simulink model "nmm2DFullBody"  (R2018a)
settings: Solver=ode23s  StartTime=0.0  StopTime=13  FixedStep=1e-3  MaxStep=ts_max  RelTol=1e-3  AbsTol=1e-4  EnableMultiTasking=on
InitFcn:
  | addpath('../lib');
  | addpath('./init_script');
  | nms_model_MechInit
  | nms_model_ControlInit
StopFcn:
  | mRFX = struct;
  | 
  | mRFX.RStance = DataFromModel.Data(:,2)
  | mRFX.RGRF_AP = DataFromModel.Data(:,24)
  | mRFX.RGRF_VT = DataFromModel.Data(:,22)
  | mRFX.RAnkleAngle = DataFromModel.Data(:,8)
  | mRFX.RKneeAngle = DataFromModel.Data(:,7)
  | mRFX.RHipAngle = DataFromModel.Data(:,6)
  | mRFX.RAnkleTorque = DataFromModel.Data(:,20)
  | mRFX.RKneeTorque = DataFromModel.Data(:,19)
  | mRFX.RHipTorque = DataFromModel.Data(:,18)
  | 
  | mRFX.RMuscleGLU = DataFromModel.Data(:,32)
  | mRFX.RMuscleHF = DataFromModel.Data(:,33)
  | mRFX.RMuscleHAM = DataFromModel.Data(:,34)
  | mRFX.RMuscleVAS = DataFromModel.Data(:,35)
  | mRFX.RMuscleGAS = DataFromModel.Data(:,36)
  | mRFX.RMuscleSOL = DataFromModel.Data(:,37)
  | mRFX.RMuscleTA = DataFromModel.Data(:,38)
  | 
  | mRFX.LStance = DataFromModel.Data(:,1)
  | mRFX.LGRF_AP = DataFromModel.Data(:,23)
  | mRFX.LGRF_VT = DataFromModel.Data(:,21)
  | mRFX.LAnkleAngle = DataFromModel.Data(:,5)
  | mRFX.LKneeAngle = DataFromModel.Data(:,4)
  | mRFX.LHipAngle = DataFromModel.Data(:,3)
  | mRFX.LAnkleTorque = DataFromModel.Data(:,17)
  | mRFX.LKneeTorque = DataFromModel.Data(:,16)
  | mRFX.LHipTorque = DataFromModel.Data(:,15)
  | 
  | mRFX.LMuscleGLU = DataFromModel.Data(:,25)
  | mRFX.LMuscleHF = DataFromModel.Data(:,26)
  | mRFX.LMuscleHAM = DataFromModel.Data(:,27)
  | mRFX.LMuscleVAS = DataFromModel.Data(:,28)
  | mRFX.LMuscleGAS = DataFromModel.Data(:,29)
  | mRFX.LMuscleSOL = DataFromModel.Data(:,30)
  | mRFX.LMuscleTA = DataFromModel.Data(:,31)
undefined symbols (not defined in the file or in its folder): alphaFmGas, alphaFmGlu, alphaFmHam, alphaFmSol, alphaFmVas, alphaLceHam, alphaLceHfl, alphaLceTa, alphaLceTa1, Amp, amp_var, c, c_jointstop, D12_F, D12_S, D12_T, D13_F, D1G_F, D1G_HAT, D1G_S, D1G_T, DeltaThRef, eref, FmaxGAS, FmaxGLU, FmaxHAM, FmaxHFL, FmaxSOL, FmaxTA, FmaxVAS, freq, freq_var, GainDeltaTheta, GainGAS, GainGLU, GainHAM, GainHAMHFL, GainHFL, GainKneOverExt, GainSOL, GainSOLTA, GainTA, GainVAS, In_F, In_HAT, In_S, In_T, K, k_gx, k_gy, k_pressure, K_swing, LceOffsetHAM, LceOffsetHFL, LceOffsetTA, LongDelay, loptGAS, loptGLU, loptHAM, loptHFL ... (+83)
libraries: nmc x77, mblibv1 x60, simulink x33, simulink_extras x18
(part 6 of 8)

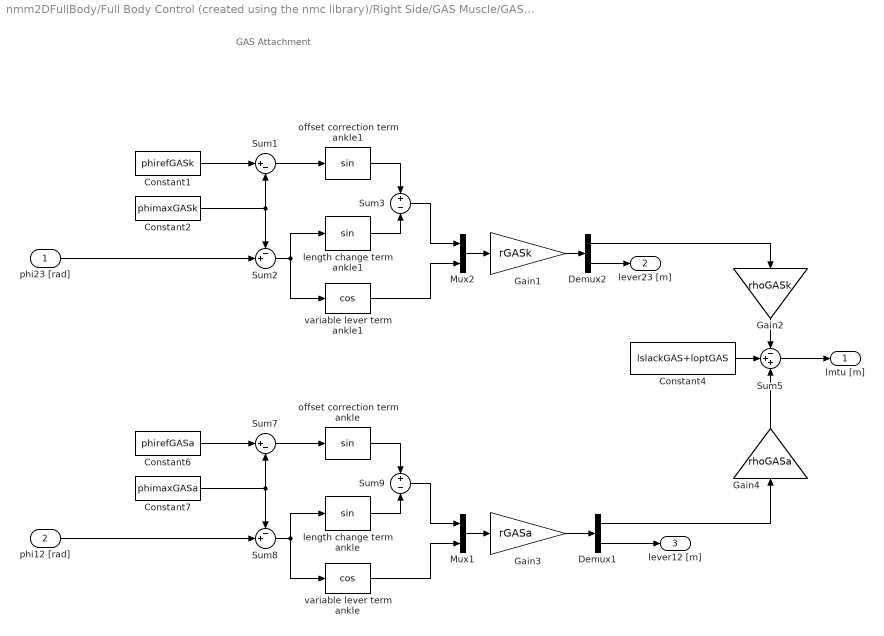
== system nmm2DFullBody/Full Body Control (created using the nmc library)/Right Side/GAS Muscle/GAS Actuation /GAS Link ==
  note: GAS Attachment
  phi23 [rad] : Inport
  phi12 [rad] : Inport  Port=2
  Constant1 : Constant  Value=phirefGASk
  Constant2 : Constant  Value=phimaxGASk
  Constant4 : Constant  Value=lslackGAS+loptGAS
  Constant6 : Constant  Value=phirefGASa
  Constant7 : Constant  Value=phimaxGASa
  Demux1 : Demux  Outputs=2
  Demux2 : Demux  Outputs=2
  Gain1 : Gain  Gain=rGASk
  Gain2 : Gain  Gain=rhoGASk
  Gain3 : Gain  Gain=rGASa
  Gain4 : Gain  Gain=rhoGASa
  Mux1 : Mux  Inputs=2
  Mux2 : Mux  Inputs=2
  Sum1 : Sum  Inputs=|+-
  Sum2 : Sum  Inputs=-+|
  Sum3 : Sum  Inputs=+-
  Sum5 : Sum  Inputs=-++
  Sum7 : Sum  Inputs=|+-
  Sum8 : Sum  Inputs=-+|
  Sum9 : Sum  Inputs=+-
  length change term ankle : Trigonometry
  length change term ankle1 : Trigonometry
  offset correction term ankle : Trigonometry
  offset correction term ankle1 : Trigonometry
  variable lever term ankle : Trigonometry  Operator=cos
  variable lever term ankle1 : Trigonometry  Operator=cos
  lmtu [m] : Outport
  lever23 [m] : Outport  Port=2
  lever12 [m] : Outport  Port=3
  wires:
  phi12 [rad]/1 -> Sum8/2
  Sum5/1 -> lmtu [m]/1
  variable lever term ankle/1 -> Mux1/2
  Demux1/2 -> lever12 [m]/1
  Sum8/1 -> variable lever term ankle/1, length change term ankle/1
  Constant7/1 -> Sum8/1, Sum7/2
  Sum7/1 -> offset correction term ankle/1
  Constant6/1 -> Sum7/1
  length change term ankle/1 -> Sum9/2
  offset correction term ankle/1 -> Sum9/1
  Sum9/1 -> Mux1/1
  Constant4/1 -> Sum5/2
  Mux1/1 -> Gain3/1
  Gain3/1 -> Demux1/1
  Demux1/1 -> Gain4/1
  Gain4/1 -> Sum5/3
  phi23 [rad]/1 -> Sum2/2
  variable lever term ankle1/1 -> Mux2/2
  Sum2/1 -> variable lever term ankle1/1, length change term ankle1/1
  Constant2/1 -> Sum2/1, Sum1/2
  Sum1/1 -> offset correction term ankle1/1
  Constant1/1 -> Sum1/1
  length change term ankle1/1 -> Sum3/2
  offset correction term ankle1/1 -> Sum3/1
  Sum3/1 -> Mux2/1
  Mux2/1 -> Gain1/1
  Gain1/1 -> Demux2/1
  Demux2/2 -> lever23 [m]/1
  Demux2/1 -> Gain2/1
  Gain2/1 -> Sum5/1

== system nmm2DFullBody/Full Body Control (created using the nmc library)/Right Side/GAS Muscle/GAS Control/ Swing Phase ==
  note: GAS Control
  note: Swing Phase Control
  Enable : EnablePort  StatesWhenEnabling=reset
  Stimulation Bias1 : Constant  Value=PreStimGAS
  StimGAS : Outport  OutputWhenDisabled=reset  InitialOutput=0
  wires:
  Stimulation Bias1/1 -> StimGAS/1

== system nmm2DFullBody/Full Body Control (created using the nmc library)/Right Side/GAS Muscle/GAS Control/Stance Phase ==
  note: GAS Control
  note: Stance Phase Control
  FmGAS : Inport
  Enable : EnablePort  StatesWhenEnabling=reset
  FB Gain2 : Gain  Gain=GainGAS  SaturateOnIntegerOverflow=on  OutDataTypeStr=Inherit: Same as input  ParamDataTypeStr=Inherit: Same as input
  Stimulation Bias1 : Constant  Value=PreStimGAS
  Sum3 : Sum  Inputs=|++  SaturateOnIntegerOverflow=on  InputSameDT=on  OutDataTypeStr=Inherit: Same as first input
  StimGAS : Outport  OutputWhenDisabled=reset  InitialOutput=0
  wires:
  FmGAS/1 -> FB Gain2/1
  Stimulation Bias1/1 -> Sum3/1
  Sum3/1 -> StimGAS/1
  FB Gain2/1 -> Sum3/2

== system nmm2DFullBody/Full Body Control (created using the nmc library)/Right Side/GLU Muscle/GLU Actuation/ GLU ==
  note: SOLEUS Muscle-Tendon Dynamics
  note: Excitation Contraction Coupling
  STIM : Inport
  lmtc [m] : Inport  Port=2
  1 : Product  Inputs=**  SaturateOnIntegerOverflow=on  InputSameDT=on  OutDataTypeStr=Inherit: Same as first input
  1/lslack : Gain  Gain=1/lslackGLU  SaturateOnIntegerOverflow=on  OutDataTypeStr=Inherit: Same as input  ParamDataTypeStr=Inherit: Same as input
  BE force-length relation : Subsystem
  CE force-length relation : Subsystem
  CE inverse force-velocity relation : Subsystem
  Constant : Constant  Value=lslackGLU
  ECC TransferFcn : simulink_extras/Additional Linear/Transfer Fcn (with initial outputs)  N=[1]  D="[tau  1]"  Y0=preA  U0=0
      settings: AttributesFormatString=pre-activation: %<Y0>
  Fmax : Gain  Gain=FmaxGLU  SaturateOnIntegerOverflow=on  OutDataTypeStr=Inherit: Same as input  ParamDataTypeStr=Inherit: Same as input
  Fv = Fse / (A*Fce) : Product  Inputs=*/  SaturateOnIntegerOverflow=on  InputSameDT=on  OutDataTypeStr=Inherit: Same as first input
  Integrator : Integrator  InitialConditionSource=external  LowerSaturationLimit=0.05
  PE force-length relation : Subsystem
  SE force-length relation : Subsystem
  Sum : Sum  Inputs=|+-  SaturateOnIntegerOverflow=on  InputSameDT=on  OutDataTypeStr=Inherit: Same as first input
  Sum2 : Sum  Inputs=|-+  SaturateOnIntegerOverflow=on  InputSameDT=on  OutDataTypeStr=Inherit: Same as first input
  Sum3 : Sum  SaturateOnIntegerOverflow=on  InputSameDT=on  OutDataTypeStr=Inherit: Same as first input
  Sum4 : Sum  SaturateOnIntegerOverflow=on  InputSameDT=on  OutDataTypeStr=Inherit: Same as first input
  lce/lopt : Gain  Gain=1/loptGLU  SaturateOnIntegerOverflow=on  OutDataTypeStr=Inherit: Same as input  ParamDataTypeStr=Inherit: Same as input
  vmax*lopt : Gain  Gain=vmaxGLU*loptGLU  SaturateOnIntegerOverflow=on  OutDataTypeStr=Inherit: Same as input  ParamDataTypeStr=Inherit: Same as input
  Fmtc : Outport  InitialOutput=0
  Lce : Outport  Port=2  InitialOutput=0
  Vce : Outport  Port=3  InitialOutput=0
  Lse : Outport  Port=4  InitialOutput=0
  A : Outport  Port=5  InitialOutput=0
  wires:
  Integrator/1 -> Sum/2, lce/lopt/1, Lce/1  "lce"
  Sum/1 -> 1/lslack/1, Lse/1  "lse"
  lce/lopt/1 -> CE force-length relation/1(lce [lopt]), BE force-length relation/1(lce [lopt]), PE force-length relation/1(lce [lopt])
  Fv = Fse / (A*Fce)/1 -> CE inverse force-velocity relation/1(Fv[Fmax])  "fv"
  vmax*lopt/1 -> Integrator/1, Vce/1  "vce"
  lmtc [m]/1 -> Sum2/2, Sum/1  "lmtc"
  Fmax/1 -> Fmtc/1  "Fmtc"
  1/lslack/1 -> SE force-length relation/1(lse [lslack])
  SE force-length relation/1(fse [Fmax]) -> Fmax/1, Sum4/1
  Sum2/1 -> Integrator/2
  Constant/1 -> Sum2/1
  CE force-length relation/1(fce [Fmax]) -> 1/1
  Sum4/1 -> Fv = Fse / (A*Fce)/1
  PE force-length relation/1(fpe [Fmax]) -> Sum3/1
  1/1 -> Sum3/2
  BE force-length relation/1(fbe [Fmax]) -> Sum4/2
  Sum3/1 -> Fv = Fse / (A*Fce)/2
  CE inverse force-velocity relation/1(v[vmax]) -> vmax*lopt/1
  STIM/1 -> ECC TransferFcn/1
  ECC TransferFcn/1 -> A/1, 1/2

== system nmm2DFullBody/Full Body Control (created using the nmc library)/Right Side/GLU Muscle/GLU Actuation/GLU Link ==
  note: GLUTEUS Attachment
  phi34 [rad] : Inport
  Constant : Constant  Value=lslackGLU+loptGLU
  Constant1 : Constant  Value=rGLU
  Constant2 : Constant  Value=phirefGLU
  Gain2 : Gain  Gain=rhoGLU
  Product : Product  RndMeth=Zero
  Sum2 : Sum  Inputs=|+-
  Sum5 : Sum  Inputs=|+-
  lmtu [m] : Outport
  lever [m] : Outport  Port=2
  wires:
  Constant/1 -> Sum5/1
  Sum5/1 -> lmtu [m]/1
  Product/1 -> Gain2/1
  phi34 [rad]/1 -> Sum2/1
  Constant2/1 -> Sum2/2
  Sum2/1 -> Product/1
  Constant1/1 -> Product/2, lever [m]/1
  Gain2/1 -> Sum5/2

== system nmm2DFullBody/Full Body Control (created using the nmc library)/Right Side/GLU Muscle/GLU Control/ Swing Phase ==
  note: Swing Phase Control
  note: GLU Control
  FmGLU : Inport
  Enable : EnablePort  StatesWhenEnabling=reset
  FB Gain2 : Gain  Gain=GainGLU  SaturateOnIntegerOverflow=on  OutDataTypeStr=Inherit: Same as input  ParamDataTypeStr=Inherit: Same as input
  Stimulation Bias3 : Constant  Value=PreStimGLU
  Sum4 : Sum  Inputs=|++  SaturateOnIntegerOverflow=on  InputSameDT=on  OutDataTypeStr=Inherit: Same as first input
  StimGLU : Outport  OutputWhenDisabled=reset  InitialOutput=0
  wires:
  FB Gain2/1 -> Sum4/2
  FmGLU/1 -> FB Gain2/1
  Stimulation Bias3/1 -> Sum4/1
  Sum4/1 -> StimGLU/1

== system nmm2DFullBody/Full Body Control (created using the nmc library)/Right Side/GLU Muscle/GLU Control/Stance Phase ==
  note: GLU Control
  note: Stance Phase Control
  note: load bearing potential
  Theta : Inport
  dTheta [rad/s] : Inport  Port=2
  CLdxThigh [N] : Inport  Port=3
  OLonCL : Inport  Port=4
  Enable : EnablePort  StatesWhenEnabling=reset
  Divide : Product
  FB Gain10 : Gain  Gain=SpeedGainGG  SaturateOnIntegerOverflow=on  OutDataTypeStr=Inherit: Same as input  ParamDataTypeStr=Inherit: Same as input
  FB Gain11 : Gain  Gain=PosGainGG  SaturateOnIntegerOverflow=on  OutDataTypeStr=Inherit: Same as input  ParamDataTypeStr=Inherit: Same as input
  FB Gain6 : Gain  Gain=1/DeltaThRef  SaturateOnIntegerOverflow=on  OutDataTypeStr=Inherit: Same as input  ParamDataTypeStr=Inherit: Same as input
  Gain1 : Gain  Gain=0.7
  Gain4 : Gain  Gain=K_swing
  Saturation2 : Saturate  UpperLimit=inf  LowerLimit=0  ZeroCross=off
  Saturation3 : Saturate  UpperLimit=1  LowerLimit=0  ZeroCross=off
  Stimulation Bias6 : Constant  Value=Theta0
  Stimulation Bias7 : Constant  Value=PreStimGG
  Sum10 : Sum  Inputs=|++  SaturateOnIntegerOverflow=on  InputSameDT=on  OutDataTypeStr=Inherit: Same as first input
  Sum12 : Sum  SaturateOnIntegerOverflow=on  InputSameDT=on  OutDataTypeStr=Inherit: Same as first input
  Sum8 : Sum  Inputs=+-  SaturateOnIntegerOverflow=on  InputSameDT=on  OutDataTypeStr=Inherit: Same as first input
  Sum9 : Sum  Inputs=|+-  SaturateOnIntegerOverflow=on  InputSameDT=on  OutDataTypeStr=Inherit: Same as first input
  positive half : Saturate  UpperLimit=inf  LowerLimit=0  ZeroCross=off
  StimGLU : Outport  OutputWhenDisabled=reset  InitialOutput=0
  wires:
  dTheta [rad/s]/1 -> FB Gain10/1
  Stimulation Bias6/1 -> Sum9/2
  Theta/1 -> Sum9/1
  Sum9/1 -> FB Gain11/1
  positive half/1 -> Sum10/2
  Stimulation Bias7/1 -> Sum10/1
  FB Gain11/1 -> Sum12/1
  FB Gain10/1 -> Sum12/2
  Sum12/1 -> positive half/1
  Saturation2/1 -> FB Gain6/1
  Sum10/1 -> Divide/1
  CLdxThigh [N]/1 -> Saturation2/1
  Gain1/1 -> StimGLU/1
  FB Gain6/1 -> Divide/2
  Divide/1 -> Saturation3/1
  Sum8/1 -> Gain1/1
  Gain4/1 -> Sum8/2
  Saturation3/1 -> Sum8/1
  OLonCL/1 -> Gain4/1

== system nmm2DFullBody/Full Body Control (created using the nmc library)/Right Side/HFL&HAM Muscles/HAM Actuation / HAM Link ==
  note: HAM Attachment
  phi34 [rad] : Inport
  phi23 [rad] : Inport  Port=2
  Constant3 : Constant  Value=rHAMh
  Constant4 : Constant  Value=lslackHAM+loptHAM
  Constant5 : Constant  Value=phirefHAMh
  Constant6 : Constant  Value=phirefHAMk
  Constant7 : Constant  Value=phimaxHAMk  VectorParams1D=off
  Demux1 : Demux  Outputs=2
  Gain2 : Gain  Gain=rhoHAMh
  Gain3 : Gain  Gain=rHAMk
  Gain4 : Gain  Gain=rhoHAMk
  Mux1 : Mux  Inputs=2
  Product : Product  RndMeth=Zero
  Sum4 : Sum  Inputs=|+-
  Sum5 : Sum  Inputs=-+-
  Sum7 : Sum  Inputs=|+-
  Sum8 : Sum  Inputs=-+|
  Sum9 : Sum  Inputs=+-
  length change term ankle : Trigonometry
  offset correction term ankle : Trigonometry
  variable lever term ankle : Trigonometry  Operator=cos
  lmtu [m] : Outport
  lever34 [m] : Outport  Port=2
  lever23 [m] : Outport  Port=3
  wires:
  phi23 [rad]/1 -> Sum8/2
  Sum5/1 -> lmtu [m]/1
  variable lever term ankle/1 -> Mux1/2
  Demux1/2 -> lever23 [m]/1
  Sum8/1 -> variable lever term ankle/1, length change term ankle/1
  Constant7/1 -> Sum8/1, Sum7/2
  Sum7/1 -> offset correction term ankle/1
  Constant6/1 -> Sum7/1
  length change term ankle/1 -> Sum9/2
  offset correction term ankle/1 -> Sum9/1
  Sum9/1 -> Mux1/1
  Constant4/1 -> Sum5/2
  Mux1/1 -> Gain3/1
  Gain3/1 -> Demux1/1
  Demux1/1 -> Gain4/1
  Gain4/1 -> Sum5/3
  Gain2/1 -> Sum5/1
  phi34 [rad]/1 -> Sum4/1
  Constant5/1 -> Sum4/2
  Sum4/1 -> Product/1
  Constant3/1 -> Product/2, lever34 [m]/1
  Product/1 -> Gain2/1

== system nmm2DFullBody/Full Body Control (created using the nmc library)/Right Side/HFL&HAM Muscles/HAM Actuation /HAM ==
  note: SOLEUS Muscle-Tendon Dynamics
  note: Excitation Contraction Coupling
  STIM : Inport
  lmtc [m] : Inport  Port=2
  1 : Product  Inputs=**  SaturateOnIntegerOverflow=on  InputSameDT=on  OutDataTypeStr=Inherit: Same as first input
  1/lslack : Gain  Gain=1/lslackHAM  SaturateOnIntegerOverflow=on  OutDataTypeStr=Inherit: Same as input  ParamDataTypeStr=Inherit: Same as input
  BE force-length relation : Subsystem
  CE force-length relation : Subsystem
  CE inverse force-velocity relation : Subsystem
  Constant : Constant  Value=lslackHAM
  ECC TransferFcn : simulink_extras/Additional Linear/Transfer Fcn (with initial outputs)  N=[1]  D="[tau  1]"  Y0=preA  U0=0
      settings: AttributesFormatString=pre-activation: %<Y0>
  Fmax : Gain  Gain=FmaxHAM  SaturateOnIntegerOverflow=on  OutDataTypeStr=Inherit: Same as input  ParamDataTypeStr=Inherit: Same as input
  Fv = Fse / (A*Fce) : Product  Inputs=*/  SaturateOnIntegerOverflow=on  InputSameDT=on  OutDataTypeStr=Inherit: Same as first input
  Integrator : Integrator  InitialConditionSource=external  LowerSaturationLimit=0.05
  PE force-length relation : Subsystem
  SE force-length relation : Subsystem
  Sum : Sum  Inputs=|+-  SaturateOnIntegerOverflow=on  InputSameDT=on  OutDataTypeStr=Inherit: Same as first input
  Sum2 : Sum  Inputs=|-+  SaturateOnIntegerOverflow=on  InputSameDT=on  OutDataTypeStr=Inherit: Same as first input
  Sum3 : Sum  SaturateOnIntegerOverflow=on  InputSameDT=on  OutDataTypeStr=Inherit: Same as first input
  Sum4 : Sum  SaturateOnIntegerOverflow=on  InputSameDT=on  OutDataTypeStr=Inherit: Same as first input
  lce/lopt : Gain  Gain=1/loptHAM  SaturateOnIntegerOverflow=on  OutDataTypeStr=Inherit: Same as input  ParamDataTypeStr=Inherit: Same as input
  vmax*lopt : Gain  Gain=vmaxHAM*loptHAM  SaturateOnIntegerOverflow=on  OutDataTypeStr=Inherit: Same as input  ParamDataTypeStr=Inherit: Same as input
  Fmtc : Outport  InitialOutput=0
  Lce : Outport  Port=2  InitialOutput=0
  Vce : Outport  Port=3  InitialOutput=0
  Lse : Outport  Port=4  InitialOutput=0
  A : Outport  Port=5  InitialOutput=0
  wires:
  Integrator/1 -> Sum/2, lce/lopt/1, Lce/1  "lce"
  Sum/1 -> 1/lslack/1, Lse/1  "lse"
  lce/lopt/1 -> CE force-length relation/1(lce [lopt]), BE force-length relation/1(lce [lopt]), PE force-length relation/1(lce [lopt])
  Fv = Fse / (A*Fce)/1 -> CE inverse force-velocity relation/1(Fv[Fmax])  "fv"
  vmax*lopt/1 -> Integrator/1, Vce/1  "vce"
  lmtc [m]/1 -> Sum2/2, Sum/1  "lmtc"
  Fmax/1 -> Fmtc/1  "Fmtc"
  1/lslack/1 -> SE force-length relation/1(lse [lslack])
  SE force-length relation/1(fse [Fmax]) -> Fmax/1, Sum4/1
  Sum2/1 -> Integrator/2
  Constant/1 -> Sum2/1
  CE force-length relation/1(fce [Fmax]) -> 1/1
  Sum4/1 -> Fv = Fse / (A*Fce)/1
  PE force-length relation/1(fpe [Fmax]) -> Sum3/1
  1/1 -> Sum3/2
  BE force-length relation/1(fbe [Fmax]) -> Sum4/2
  Sum3/1 -> Fv = Fse / (A*Fce)/2
  CE inverse force-velocity relation/1(v[vmax]) -> vmax*lopt/1
  STIM/1 -> ECC TransferFcn/1
  ECC TransferFcn/1 -> 1/2, A/1

== system nmm2DFullBody/Full Body Control (created using the nmc library)/Right Side/HFL&HAM Muscles/HFL Actuation/ HFL ==
  note: SOLEUS Muscle-Tendon Dynamics
  note: Excitation Contraction Coupling
  STIM : Inport
  lmtc [m] : Inport  Port=2
  1 : Product  Inputs=**  SaturateOnIntegerOverflow=on  InputSameDT=on  OutDataTypeStr=Inherit: Same as first input
  1/lslack : Gain  Gain=1/lslackHFL  SaturateOnIntegerOverflow=on  OutDataTypeStr=Inherit: Same as input  ParamDataTypeStr=Inherit: Same as input
  BE force-length relation : Subsystem
  CE force-length relation : Subsystem
  CE inverse force-velocity relation : Subsystem
  Constant : Constant  Value=lslackHFL
  ECC TransferFcn : simulink_extras/Additional Linear/Transfer Fcn (with initial outputs)  N=[1]  D="[tau  1]"  Y0=preA  U0=0
      settings: AttributesFormatString=pre-activation: %<Y0>
  Fmax : Gain  Gain=FmaxHFL  SaturateOnIntegerOverflow=on  OutDataTypeStr=Inherit: Same as input  ParamDataTypeStr=Inherit: Same as input
  Fv = Fse / (A*Fce) : Product  Inputs=*/  SaturateOnIntegerOverflow=on  InputSameDT=on  OutDataTypeStr=Inherit: Same as first input
  Integrator : Integrator  InitialConditionSource=external  LowerSaturationLimit=0.05
  PE force-length relation : Subsystem
  SE force-length relation : Subsystem
  Sum : Sum  Inputs=|+-  SaturateOnIntegerOverflow=on  InputSameDT=on  OutDataTypeStr=Inherit: Same as first input
  Sum2 : Sum  Inputs=|-+  SaturateOnIntegerOverflow=on  InputSameDT=on  OutDataTypeStr=Inherit: Same as first input
  Sum3 : Sum  SaturateOnIntegerOverflow=on  InputSameDT=on  OutDataTypeStr=Inherit: Same as first input
  Sum4 : Sum  SaturateOnIntegerOverflow=on  InputSameDT=on  OutDataTypeStr=Inherit: Same as first input
  lce/lopt : Gain  Gain=1/loptHFL  SaturateOnIntegerOverflow=on  OutDataTypeStr=Inherit: Same as input  ParamDataTypeStr=Inherit: Same as input
  vmax*lopt : Gain  Gain=vmaxHFL*loptHFL  SaturateOnIntegerOverflow=on  OutDataTypeStr=Inherit: Same as input  ParamDataTypeStr=Inherit: Same as input
  Fmtc : Outport  InitialOutput=0
  Lce : Outport  Port=2  InitialOutput=0
  Vce : Outport  Port=3  InitialOutput=0
  Lse : Outport  Port=4  InitialOutput=0
  A : Outport  Port=5  InitialOutput=0
  wires:
  Integrator/1 -> Sum/2, lce/lopt/1, Lce/1  "lce"
  Sum/1 -> 1/lslack/1, Lse/1  "lse"
  lce/lopt/1 -> CE force-length relation/1(lce [lopt]), BE force-length relation/1(lce [lopt]), PE force-length relation/1(lce [lopt])
  Fv = Fse / (A*Fce)/1 -> CE inverse force-velocity relation/1(Fv[Fmax])  "fv"
  vmax*lopt/1 -> Integrator/1, Vce/1  "vce"
  lmtc [m]/1 -> Sum2/2, Sum/1  "lmtc"
  Fmax/1 -> Fmtc/1  "Fmtc"
  1/lslack/1 -> SE force-length relation/1(lse [lslack])
  SE force-length relation/1(fse [Fmax]) -> Fmax/1, Sum4/1
  Sum2/1 -> Integrator/2
  Constant/1 -> Sum2/1
  CE force-length relation/1(fce [Fmax]) -> 1/1
  Sum4/1 -> Fv = Fse / (A*Fce)/1
  PE force-length relation/1(fpe [Fmax]) -> Sum3/1
  1/1 -> Sum3/2
  BE force-length relation/1(fbe [Fmax]) -> Sum4/2
  Sum3/1 -> Fv = Fse / (A*Fce)/2
  CE inverse force-velocity relation/1(v[vmax]) -> vmax*lopt/1
  STIM/1 -> ECC TransferFcn/1
  ECC TransferFcn/1 -> A/1, 1/2

== system nmm2DFullBody/Full Body Control (created using the nmc library)/Right Side/HFL&HAM Muscles/HFL Actuation/ HFL Link ==
  note: HFL Attachment
  phi34 [rad] : Inport
  Constant : Constant  Value=lslackHFL+loptHFL
  Constant1 : Constant  Value=rHFL
  Constant2 : Constant  Value=phirefHFL
  Gain2 : Gain  Gain=rhoHFL
  Product : Product  RndMeth=Zero
  Sum2 : Sum  Inputs=|+-
  Sum5 : Sum  Inputs=|++
  lmtu [m] : Outport
  lever [m] : Outport  Port=2
  wires:
  Constant/1 -> Sum5/1
  Sum5/1 -> lmtu [m]/1
  Product/1 -> Gain2/1
  phi34 [rad]/1 -> Sum2/1
  Constant2/1 -> Sum2/2
  Sum2/1 -> Product/1
  Constant1/1 -> Product/2, lever [m]/1
  Gain2/1 -> Sum5/2

== system nmm2DFullBody/Full Body Control (created using the nmc library)/Right Side/HFL&HAM Muscles/HFL&HAM Control/Stance Phase ==
  note: Stance Phase Control
  note: HAM Control
  note: cross leg influence
  note: HFL Control
  note: load bearing potential
  Theta : Inport
  dTheta [rad/s] : Inport  Port=2
  CLdxThigh [N] : Inport  Port=3
  OLonCL : Inport  Port=4
  Enable : EnablePort  StatesWhenEnabling=reset
  Divide : Product
  Divide1 : Product
  FB Gain10 : Gain  Gain=SpeedGainGG  SaturateOnIntegerOverflow=on  OutDataTypeStr=Inherit: Same as input  ParamDataTypeStr=Inherit: Same as input
  FB Gain11 : Gain  Gain=PosGainGG  SaturateOnIntegerOverflow=on  OutDataTypeStr=Inherit: Same as input  ParamDataTypeStr=Inherit: Same as input
  FB Gain6 : Gain  Gain=1/DeltaThRef  SaturateOnIntegerOverflow=on  OutDataTypeStr=Inherit: Same as input  ParamDataTypeStr=Inherit: Same as input
  Gain : Gain
  Gain3 : Gain  Gain=K_swing
  Saturation1 : Saturate  UpperLimit=1  LowerLimit=0  ZeroCross=off
  Saturation2 : Saturate  UpperLimit=inf  LowerLimit=0  ZeroCross=off
  Saturation3 : Saturate  UpperLimit=1  LowerLimit=0  ZeroCross=off
  Stimulation Bias6 : Constant  Value=Theta0
  Stimulation Bias7 : Constant  Value=PreStimGG
  Sum10 : Sum  Inputs=|++  SaturateOnIntegerOverflow=on  InputSameDT=on  OutDataTypeStr=Inherit: Same as first input
  Sum11 : Sum  Inputs=-+|  SaturateOnIntegerOverflow=on  InputSameDT=on  OutDataTypeStr=Inherit: Same as first input
  Sum12 : Sum  SaturateOnIntegerOverflow=on  InputSameDT=on  OutDataTypeStr=Inherit: Same as first input
  Sum13 : Sum  SaturateOnIntegerOverflow=on  InputSameDT=on  OutDataTypeStr=Inherit: Same as first input
  Sum9 : Sum  Inputs=|+-  SaturateOnIntegerOverflow=on  InputSameDT=on  OutDataTypeStr=Inherit: Same as first input
  negative half : Saturate  UpperLimit=0  LowerLimit=-inf  ZeroCross=off
  positive half : Saturate  UpperLimit=inf  LowerLimit=0  ZeroCross=off
  StimHFL : Outport  OutputWhenDisabled=reset  InitialOutput=0
  StimHAM : Outport  Port=2  OutputWhenDisabled=reset  InitialOutput=0
  Delta_Theta : Outport  Port=3  InitialOutput=0
  wires:
  dTheta [rad/s]/1 -> FB Gain10/1
  Stimulation Bias6/1 -> Sum9/2
  Theta/1 -> Sum9/1
  negative half/1 -> Sum11/1
  Sum9/1 -> FB Gain11/1, Delta_Theta/1
  positive half/1 -> Sum10/2
  Stimulation Bias7/1 -> Sum10/1, Sum11/2
  FB Gain11/1 -> Sum12/1
  FB Gain10/1 -> Sum12/2
  Sum12/1 -> positive half/1, negative half/1
  Sum13/1 -> StimHFL/1
  Saturation1/1 -> Sum13/1
  Saturation2/1 -> FB Gain6/1
  Sum11/1 -> Divide1/2
  Sum10/1 -> Divide/1
  CLdxThigh [N]/1 -> Saturation2/1
  Divide1/1 -> Saturation1/1
  Gain3/1 -> Sum13/2
  FB Gain6/1 -> Divide/2, Divide1/1
  Divide/1 -> Saturation3/1
  Saturation3/1 -> Gain/1
  OLonCL/1 -> Gain3/1
  Gain/1 -> StimHAM/1

== system nmm2DFullBody/Full Body Control (created using the nmc library)/Right Side/HFL&HAM Muscles/HFL&HAM Control/Swing Phase ==
  note: Swing Phase Control
  note: HAM Control
  note: HFL Control
  Delta_Theta : Inport
  LceHFL : Inport  Port=2
  LceHAM : Inport  Port=3
  FmHAM : Inport  Port=4
  Enable : EnablePort  StatesWhenEnabling=reset
  FB Gain1 : Gain  Gain=GainHAM  SaturateOnIntegerOverflow=on  OutDataTypeStr=Inherit: Same as input  ParamDataTypeStr=Inherit: Same as input
  L+: 0.18 F+: 0.9/Fmax : Gain  Gain=GainHFL  SaturateOnIntegerOverflow=on  OutDataTypeStr=Inherit: Same as input  ParamDataTypeStr=Inherit: Same as input
  L+: 2 : Gain  Gain=GainDeltaTheta  SaturateOnIntegerOverflow=on  OutDataTypeStr=Inherit: Same as input  ParamDataTypeStr=Inherit: Same as input
  L+: 3 : Gain  Gain=GainHAMHFL  SaturateOnIntegerOverflow=on  OutDataTypeStr=Inherit: Same as input  ParamDataTypeStr=Inherit: Same as input
  Stimulation Bias4 : Constant  Value=PreStimHAM
  Sum12 : Sum  Inputs=|+-  SaturateOnIntegerOverflow=on  InputSameDT=on  OutDataTypeStr=Inherit: Same as first input
  Sum2 : Sum  SaturateOnIntegerOverflow=on  InputSameDT=on  OutDataTypeStr=Inherit: Same as first input
  Sum3 : Sum  Inputs=|++  SaturateOnIntegerOverflow=on  InputSameDT=on  OutDataTypeStr=Inherit: Same as first input
  Sum6 : Sum  Inputs=|++  SaturateOnIntegerOverflow=on  InputSameDT=on  OutDataTypeStr=Inherit: Same as first input
  d : Constant  Value=PreStimHFL
  StimHFL : Outport  OutputWhenDisabled=reset  InitialOutput=0
  StimHAM : Outport  Port=2  OutputWhenDisabled=reset  InitialOutput=0
  wires:
  FB Gain1/1 -> Sum3/2
  Stimulation Bias4/1 -> Sum3/1
  Sum3/1 -> StimHAM/1
  LceHFL/1 -> L+: 0.18 F+: 0.9/Fmax/1
  L+: 0.18 F+: 0.9/Fmax/1 -> Sum6/2
  LceHAM/1 -> L+: 3/1
  L+: 3/1 -> Sum12/2
  Sum6/1 -> Sum12/1
  Delta_Theta/1 -> L+: 2/1
  d/1 -> Sum2/1
  Sum2/1 -> Sum6/1
  L+: 2/1 -> Sum2/2
  FmHAM/1 -> FB Gain1/1
  Sum12/1 -> StimHFL/1

== system nmm2DFullBody/Full Body Control (created using the nmc library)/Right Side/SOL&TA Muscles/SOL Actuation/ SOL ==
  note: SOLEUS Muscle-Tendon Dynamics
  note: Excitation Contraction Coupling
  STIM : Inport
  lmtc [m] : Inport  Port=2
  1 : Product  Inputs=**  SaturateOnIntegerOverflow=on  InputSameDT=on  OutDataTypeStr=Inherit: Same as first input
  1/lslack : Gain  Gain=1/lslackSOL  SaturateOnIntegerOverflow=on  OutDataTypeStr=Inherit: Same as input  ParamDataTypeStr=Inherit: Same as input
  BE force-length relation : Subsystem
  CE force-length relation : Subsystem
  CE inverse force-velocity relation : Subsystem
  Constant : Constant  Value=lslackSOL
  ECC TransferFcn : simulink_extras/Additional Linear/Transfer Fcn (with initial outputs)  N=[1]  D="[tau  1]"  Y0=preA  U0=0
      settings: AttributesFormatString=pre-activation: %<Y0>
  Fmax : Gain  Gain=FmaxSOL  SaturateOnIntegerOverflow=on  OutDataTypeStr=Inherit: Same as input  ParamDataTypeStr=Inherit: Same as input
  Fv = Fse / (A*Fce) : Product  Inputs=*/  SaturateOnIntegerOverflow=on  InputSameDT=on  OutDataTypeStr=Inherit: Same as first input
  Integrator : Integrator  InitialConditionSource=external  LowerSaturationLimit=0.05
  PE force-length relation : Subsystem
  SE force-length relation : Subsystem
  Sum : Sum  Inputs=|+-  SaturateOnIntegerOverflow=on  InputSameDT=on  OutDataTypeStr=Inherit: Same as first input
  Sum2 : Sum  Inputs=|-+  SaturateOnIntegerOverflow=on  InputSameDT=on  OutDataTypeStr=Inherit: Same as first input
  Sum3 : Sum  SaturateOnIntegerOverflow=on  InputSameDT=on  OutDataTypeStr=Inherit: Same as first input
  Sum4 : Sum  SaturateOnIntegerOverflow=on  InputSameDT=on  OutDataTypeStr=Inherit: Same as first input
  lce/lopt : Gain  Gain=1/loptSOL  SaturateOnIntegerOverflow=on  OutDataTypeStr=Inherit: Same as input  ParamDataTypeStr=Inherit: Same as input
  vmax*lopt : Gain  Gain=vmaxSOL*loptSOL  SaturateOnIntegerOverflow=on  OutDataTypeStr=Inherit: Same as input  ParamDataTypeStr=Inherit: Same as input
  Fmtc : Outport  InitialOutput=0
  Lce : Outport  Port=2  InitialOutput=0
  Vce : Outport  Port=3  InitialOutput=0
  Lse : Outport  Port=4  InitialOutput=0
  A : Outport  Port=5  InitialOutput=0
  wires:
  Integrator/1 -> Sum/2, lce/lopt/1, Lce/1  "lce"
  Sum/1 -> 1/lslack/1, Lse/1  "lse"
  lce/lopt/1 -> CE force-length relation/1(lce [lopt]), BE force-length relation/1(lce [lopt]), PE force-length relation/1(lce [lopt])
  Fv = Fse / (A*Fce)/1 -> CE inverse force-velocity relation/1(Fv[Fmax])  "fv"
  vmax*lopt/1 -> Integrator/1, Vce/1  "vce"
  lmtc [m]/1 -> Sum2/2, Sum/1  "lmtc"
  Fmax/1 -> Fmtc/1  "Fmtc"
  1/lslack/1 -> SE force-length relation/1(lse [lslack])
  SE force-length relation/1(fse [Fmax]) -> Fmax/1, Sum4/1
  Sum2/1 -> Integrator/2
  Constant/1 -> Sum2/1
  CE force-length relation/1(fce [Fmax]) -> 1/1
  Sum4/1 -> Fv = Fse / (A*Fce)/1
  PE force-length relation/1(fpe [Fmax]) -> Sum3/1
  1/1 -> Sum3/2
  BE force-length relation/1(fbe [Fmax]) -> Sum4/2
  Sum3/1 -> Fv = Fse / (A*Fce)/2
  CE inverse force-velocity relation/1(v[vmax]) -> vmax*lopt/1
  STIM/1 -> ECC TransferFcn/1
  ECC TransferFcn/1 -> A/1, 1/2

== system nmm2DFullBody/Full Body Control (created using the nmc library)/Right Side/SOL&TA Muscles/SOL Actuation/SOL Link ==
  note: Soleus Attachment
  phi12 [rad] : Inport
  Constant : Constant  Value=lslackSOL+loptSOL
  Constant2 : Constant  Value=phirefSOL
  Constant3 : Constant  Value=phimaxSOL
  Demux : Demux  Outputs=2
  Gain2 : Gain  Gain=rSOL
  Gain4 : Gain  Gain=rhoSOL
  Mux : Mux  Inputs=2
  Sum2 : Sum  Inputs=|+-
  Sum3 : Sum  Inputs=-+|
  Sum4 : Sum  Inputs=+-
  Sum5 : Sum  Inputs=|++
  length change term : Trigonometry
  offset correction term : Trigonometry
  variable lever term : Trigonometry  Operator=cos
  lmtc [m] : Outport
  lever [m] : Outport  Port=2
  wires:
  phi12 [rad]/1 -> Sum3/2
  Sum3/1 -> variable lever term/1, length change term/1
  Constant3/1 -> Sum3/1, Sum2/2
  Sum2/1 -> offset correction term/1
  Constant2/1 -> Sum2/1
  length change term/1 -> Sum4/2
  offset correction term/1 -> Sum4/1
  Sum4/1 -> Mux/1
  Constant/1 -> Sum5/1
  Sum5/1 -> lmtc [m]/1
  Gain4/1 -> Sum5/2
  variable lever term/1 -> Mux/2
  Mux/1 -> Gain2/1
  Gain2/1 -> Demux/1
  Demux/1 -> Gain4/1
  Demux/2 -> lever [m]/1

== system nmm2DFullBody/Full Body Control (created using the nmc library)/Right Side/SOL&TA Muscles/SOL&TA Control/ Stance Phase ==
  note: SOL Control
  note: TA Control
  note: Stance Phase Control
  FmSOL : Inport
  LceTA : Inport  Port=2
  Enable : EnablePort  StatesWhenEnabling=reset
  FB Gain3 : Gain  Gain=GainSOLTA  SaturateOnIntegerOverflow=on  OutDataTypeStr=Inherit: Same as input  ParamDataTypeStr=Inherit: Same as input
  FB Gain4 : Gain  Gain=GainSOL  SaturateOnIntegerOverflow=on  OutDataTypeStr=Inherit: Same as input  ParamDataTypeStr=Inherit: Same as input
  FB Gain8 : Gain  Gain=GainTA  SaturateOnIntegerOverflow=on  OutDataTypeStr=Inherit: Same as input  ParamDataTypeStr=Inherit: Same as input
  Stimulation Bias2 : Constant  Value=PreStimTA
  Stimulation Bias3 : Constant  Value=PreStimSOL
  Sum4 : Sum  Inputs=|+-  SaturateOnIntegerOverflow=on  InputSameDT=on  OutDataTypeStr=Inherit: Same as first input
  Sum6 : Sum  Inputs=|++  SaturateOnIntegerOverflow=on  InputSameDT=on  OutDataTypeStr=Inherit: Same as first input
  Sum7 : Sum  Inputs=|++  SaturateOnIntegerOverflow=on  InputSameDT=on  OutDataTypeStr=Inherit: Same as first input
  StimTA : Outport  OutputWhenDisabled=reset  InitialOutput=0
  StimSOL : Outport  Port=2  OutputWhenDisabled=reset  InitialOutput=0
  wires:
  FmSOL/1 -> FB Gain4/1, FB Gain3/1
  FB Gain4/1 -> Sum6/2
  Sum6/1 -> StimSOL/1
  FB Gain3/1 -> Sum4/2
  Stimulation Bias2/1 -> Sum4/1
  Sum4/1 -> Sum7/1
  Sum7/1 -> StimTA/1
  FB Gain8/1 -> Sum7/2
  LceTA/1 -> FB Gain8/1
  Stimulation Bias3/1 -> Sum6/1

== system nmm2DFullBody/Full Body Control (created using the nmc library)/Right Side/SOL&TA Muscles/SOL&TA Control/Swing Phase ==
  note: SOL Control
  note: Swing Phase Control
  note: TA Control
  LceTA : Inport
  Enable : EnablePort  StatesWhenEnabling=reset
  Gain1 : Gain  Gain=GainTA
  Stimulation Bias2 : Constant  Value=PreStimSOL
  Stimulation Bias7 : Constant  Value=PreStimTA
  Sum1 : Sum  Inputs=|++  SaturateOnIntegerOverflow=on  InputSameDT=on  OutDataTypeStr=Inherit: Same as first input
  StimTA : Outport  OutputWhenDisabled=reset  InitialOutput=0
  StimSOL : Outport  Port=2  OutputWhenDisabled=reset  InitialOutput=0
  wires:
  Stimulation Bias2/1 -> StimSOL/1
  LceTA/1 -> Gain1/1
  Stimulation Bias7/1 -> Sum1/1
  Sum1/1 -> StimTA/1
  Gain1/1 -> Sum1/2

== system nmm2DFullBody/Full Body Control (created using the nmc library)/Right Side/SOL&TA Muscles/TA Actuation/TA ==
  note: Excitation Contraction Coupling
  note: SOLEUS Muscle-Tendon Dynamics
  STIM : Inport
  lmtc [m] : Inport  Port=2
  1 : Product  Inputs=**  SaturateOnIntegerOverflow=on  InputSameDT=on  OutDataTypeStr=Inherit: Same as first input
  1/lslack : Gain  Gain=1/lslackTA  SaturateOnIntegerOverflow=on  OutDataTypeStr=Inherit: Same as input  ParamDataTypeStr=Inherit: Same as input
  BE force-length relation : Subsystem
  CE force-length relation : Subsystem
  CE inverse force-velocity relation : Subsystem
  Constant : Constant  Value=lslackTA
  ECC TransferFcn : simulink_extras/Additional Linear/Transfer Fcn (with initial outputs)  N=[1]  D="[tau  1]"  Y0=preA  U0=0
      settings: AttributesFormatString=pre-activation: %<Y0>
  Fmax : Gain  Gain=FmaxTA  SaturateOnIntegerOverflow=on  OutDataTypeStr=Inherit: Same as input  ParamDataTypeStr=Inherit: Same as input
  Fv = Fse / (A*Fce) : Product  Inputs=*/  SaturateOnIntegerOverflow=on  InputSameDT=on  OutDataTypeStr=Inherit: Same as first input
  Integrator : Integrator  InitialConditionSource=external  LowerSaturationLimit=0.05
  PE force-length relation : Subsystem
  SE force-length relation : Subsystem
  Sum : Sum  Inputs=|+-  SaturateOnIntegerOverflow=on  InputSameDT=on  OutDataTypeStr=Inherit: Same as first input
  Sum2 : Sum  Inputs=|-+  SaturateOnIntegerOverflow=on  InputSameDT=on  OutDataTypeStr=Inherit: Same as first input
  Sum3 : Sum  SaturateOnIntegerOverflow=on  InputSameDT=on  OutDataTypeStr=Inherit: Same as first input
  Sum4 : Sum  SaturateOnIntegerOverflow=on  InputSameDT=on  OutDataTypeStr=Inherit: Same as first input
  lce/lopt : Gain  Gain=1/loptTA  SaturateOnIntegerOverflow=on  OutDataTypeStr=Inherit: Same as input  ParamDataTypeStr=Inherit: Same as input
  vmax*lopt : Gain  Gain=vmaxTA*loptTA  SaturateOnIntegerOverflow=on  OutDataTypeStr=Inherit: Same as input  ParamDataTypeStr=Inherit: Same as input
  Fmtc : Outport  InitialOutput=0
  Lce : Outport  Port=2  InitialOutput=0
  Vce : Outport  Port=3  InitialOutput=0
  Lse : Outport  Port=4  InitialOutput=0
  A : Outport  Port=5  InitialOutput=0
  wires:
  CE inverse force-velocity relation/1(v[vmax]) -> vmax*lopt/1
  Sum3/1 -> Fv = Fse / (A*Fce)/2
  BE force-length relation/1(fbe [Fmax]) -> Sum4/2
  1/1 -> Sum3/2
  PE force-length relation/1(fpe [Fmax]) -> Sum3/1
  Sum4/1 -> Fv = Fse / (A*Fce)/1
  CE force-length relation/1(fce [Fmax]) -> 1/1
  Constant/1 -> Sum2/1
  Sum2/1 -> Integrator/2
  SE force-length relation/1(fse [Fmax]) -> Sum4/1, Fmax/1
  1/lslack/1 -> SE force-length relation/1(lse [lslack])
  Fmax/1 -> Fmtc/1  "Fmtc"
  lmtc [m]/1 -> Sum/1, Sum2/2  "lmtc"
  vmax*lopt/1 -> Integrator/1, Vce/1  "vce"
  Fv = Fse / (A*Fce)/1 -> CE inverse force-velocity relation/1(Fv[Fmax])  "fv"
  lce/lopt/1 -> BE force-length relation/1(lce [lopt]), PE force-length relation/1(lce [lopt]), CE force-length relation/1(lce [lopt])
  Sum/1 -> Lse/1, 1/lslack/1  "lse"
  Integrator/1 -> lce/lopt/1, Sum/2, Lce/1  "lce"
  STIM/1 -> ECC TransferFcn/1
  ECC TransferFcn/1 -> 1/2, A/1

== system nmm2DFullBody/Full Body Control (created using the nmc library)/Right Side/SOL&TA Muscles/TA Actuation/TA Link ==
  note: Muscle Length and Moment Arm
  phi12 [rad] : Inport
  Constant : Constant  Value=lslackTA+loptTA
  Constant2 : Constant  Value=phirefTA
  Constant3 : Constant  Value=phimaxTA
  Demux : Demux  Outputs=2
  Gain2 : Gain  Gain=rTA
  Gain4 : Gain  Gain=rhoTA
  Mux : Mux  Inputs=2
  Sum2 : Sum  Inputs=|+-
  Sum3 : Sum  Inputs=-+|
  Sum4 : Sum  Inputs=+-
  Sum5 : Sum  Inputs=|+-
  length change term : Trigonometry
  offset correction term : Trigonometry
  variable lever term : Trigonometry  Operator=cos
  lmtc [m] : Outport
  lever [m] : Outport  Port=2
  wires:
  phi12 [rad]/1 -> Sum3/2
  Sum3/1 -> variable lever term/1, length change term/1
  Constant3/1 -> Sum3/1, Sum2/2
  Sum2/1 -> offset correction term/1
  Constant2/1 -> Sum2/1
  length change term/1 -> Sum4/2
  offset correction term/1 -> Sum4/1
  Sum4/1 -> Mux/1
  Constant/1 -> Sum5/1
  Sum5/1 -> lmtc [m]/1
  Gain4/1 -> Sum5/2
  variable lever term/1 -> Mux/2
  Mux/1 -> Gain2/1
  Gain2/1 -> Demux/1
  Demux/1 -> Gain4/1
  Demux/2 -> lever [m]/1

== system nmm2DFullBody/Full Body Control (created using the nmc library)/Right Side/VAS Muscle/VAS Actuation /VAS ==
  note: VASTI Muscle-Tendon Dynamics
  note: Excitation Contraction Coupling
  STIM : Inport
  lmtc [m] : Inport  Port=2
  1 : Product  Inputs=**  SaturateOnIntegerOverflow=on  InputSameDT=on  OutDataTypeStr=Inherit: Same as first input
  1/lslack : Gain  Gain=1/lslackVAS  SaturateOnIntegerOverflow=on  OutDataTypeStr=Inherit: Same as input  ParamDataTypeStr=Inherit: Same as input
  BE force-length relation : Subsystem
  CE force-length relation : Subsystem
  CE inverse force-velocity relation : Subsystem
  Constant : Constant  Value=lslackVAS
  ECC TransferFcn : simulink_extras/Additional Linear/Transfer Fcn (with initial outputs)  N=[1]  D="[tau  1]"  Y0=preA  U0=0
      settings: AttributesFormatString=pre-activation: %<Y0>
  Fmax : Gain  Gain=FmaxVAS  SaturateOnIntegerOverflow=on  OutDataTypeStr=Inherit: Same as input  ParamDataTypeStr=Inherit: Same as input
  Fv = Fse / (A*Fce) : Product  Inputs=*/  SaturateOnIntegerOverflow=on  InputSameDT=on  OutDataTypeStr=Inherit: Same as first input
  Integrator : Integrator  InitialConditionSource=external  LowerSaturationLimit=0.05
  PE force-length relation : Subsystem
  SE force-length relation : Subsystem
  Sum : Sum  Inputs=|+-  SaturateOnIntegerOverflow=on  InputSameDT=on  OutDataTypeStr=Inherit: Same as first input
  Sum2 : Sum  Inputs=|-+  SaturateOnIntegerOverflow=on  InputSameDT=on  OutDataTypeStr=Inherit: Same as first input
  Sum3 : Sum  SaturateOnIntegerOverflow=on  InputSameDT=on  OutDataTypeStr=Inherit: Same as first input
  Sum4 : Sum  SaturateOnIntegerOverflow=on  InputSameDT=on  OutDataTypeStr=Inherit: Same as first input
  lce/lopt : Gain  Gain=1/loptVAS  SaturateOnIntegerOverflow=on  OutDataTypeStr=Inherit: Same as input  ParamDataTypeStr=Inherit: Same as input
  vmax*lopt : Gain  Gain=vmaxVAS*loptVAS  SaturateOnIntegerOverflow=on  OutDataTypeStr=Inherit: Same as input  ParamDataTypeStr=Inherit: Same as input
  Fmtc : Outport  InitialOutput=0
  Lce : Outport  Port=2  InitialOutput=0
  Vce : Outport  Port=3  InitialOutput=0
  Lse : Outport  Port=4  InitialOutput=0
  A : Outport  Port=5  InitialOutput=0
  wires:
  Integrator/1 -> Sum/2, lce/lopt/1, Lce/1  "lce"
  Sum/1 -> 1/lslack/1, Lse/1  "lse"
  lce/lopt/1 -> CE force-length relation/1(lce [lopt]), BE force-length relation/1(lce [lopt]), PE force-length relation/1(lce [lopt])
  Fv = Fse / (A*Fce)/1 -> CE inverse force-velocity relation/1(Fv[Fmax])  "fv"
  vmax*lopt/1 -> Integrator/1, Vce/1  "vce"
  lmtc [m]/1 -> Sum2/2, Sum/1  "lmtc"
  Fmax/1 -> Fmtc/1  "Fmtc"
  1/lslack/1 -> SE force-length relation/1(lse [lslack])
  SE force-length relation/1(fse [Fmax]) -> Fmax/1, Sum4/1
  Sum2/1 -> Integrator/2
  Constant/1 -> Sum2/1
  CE force-length relation/1(fce [Fmax]) -> 1/1
  Sum4/1 -> Fv = Fse / (A*Fce)/1
  PE force-length relation/1(fpe [Fmax]) -> Sum3/1
  1/1 -> Sum3/2
  BE force-length relation/1(fbe [Fmax]) -> Sum4/2
  Sum3/1 -> Fv = Fse / (A*Fce)/2
  CE inverse force-velocity relation/1(v[vmax]) -> vmax*lopt/1
  STIM/1 -> ECC TransferFcn/1
  ECC TransferFcn/1 -> 1/2, A/1

== system nmm2DFullBody/Full Body Control (created using the nmc library)/Right Side/VAS Muscle/VAS Actuation /VAS Link ==
  note: Muscle Length and Moment Arm
  phi23 [rad] : Inport
  Constant : Constant  Value=lslackVAS+loptVAS
  Constant2 : Constant  Value=phirefVAS
  Constant3 : Constant  Value=phimaxVAS
  Demux : Demux  Outputs=2
  Gain2 : Gain  Gain=rVAS
  Gain4 : Gain  Gain=rhoVAS
  Mux : Mux  Inputs=2
  Sum2 : Sum  Inputs=|+-
  Sum3 : Sum  Inputs=-+|
  Sum4 : Sum  Inputs=+-
  Sum5 : Sum  Inputs=|++
  length change term : Trigonometry
  offset correction term : Trigonometry
  variable lever term : Trigonometry  Operator=cos
  lmtu [m] : Outport
  lever [m] : Outport  Port=2
  wires:
  phi23 [rad]/1 -> Sum3/2
  Sum3/1 -> variable lever term/1, length change term/1
  Constant3/1 -> Sum3/1, Sum2/2
  Sum2/1 -> offset correction term/1
  Constant2/1 -> Sum2/1
  length change term/1 -> Sum4/2
  offset correction term/1 -> Sum4/1
  Sum4/1 -> Mux/1
  Constant/1 -> Sum5/1
  Sum5/1 -> lmtu [m]/1
  Gain4/1 -> Sum5/2
  variable lever term/1 -> Mux/2
  Mux/1 -> Gain2/1
  Gain2/1 -> Demux/1
  Demux/1 -> Gain4/1
  Demux/2 -> lever [m]/1

== system nmm2DFullBody/Full Body Control (created using the nmc library)/Right Side/VAS Muscle/VAS Control/ Swing Phase ==
  note: VAS Control
  note: Swing Phase Control
  Enable : EnablePort  StatesWhenEnabling=reset
  Stimulation Bias5 : Constant  Value=0
  StimVAS : Outport  OutputWhenDisabled=reset  InitialOutput=0
  wires:
  Stimulation Bias5/1 -> StimVAS/1

== system nmm2DFullBody/Full Body Control (created using the nmc library)/Right Side/VAS Muscle/VAS Control/Stance Phase ==
  note: VAS Control
  note: Stance Phase Control
  CLKneeState : Inport
  OLonCL : Inport  Port=2
  OLdxThigh [N] : Inport  Port=3
  FmVAS : Inport  Port=4
  Enable : EnablePort  StatesWhenEnabling=reset
  FB Gain : Gain  Gain=GainVAS  SaturateOnIntegerOverflow=on  OutDataTypeStr=Inherit: Same as input  ParamDataTypeStr=Inherit: Same as input
  FB Gain1 : Gain  Gain=1/DeltaThRef  SaturateOnIntegerOverflow=on  OutDataTypeStr=Inherit: Same as input  ParamDataTypeStr=Inherit: Same as input
  Gain2 : Gain  Gain=GainKneOverExt
  Product1 : Product  RndMeth=Zero
  Saturation4 : Saturate  UpperLimit=inf  LowerLimit=0  ZeroCross=off
  Stimulation Bias : Constant  Value=PreStimVAS
  Sum1 : Sum  Inputs=-+|  SaturateOnIntegerOverflow=on  InputSameDT=on  OutDataTypeStr=Inherit: Same as first input
  Sum14 : Sum  Inputs=|+-  SaturateOnIntegerOverflow=on  InputSameDT=on  OutDataTypeStr=Inherit: Same as first input
  Sum2 : Sum  Inputs=|++  SaturateOnIntegerOverflow=on  InputSameDT=on  OutDataTypeStr=Inherit: Same as first input
  StimVAS : Outport  OutputWhenDisabled=reset  InitialOutput=0
  wires:
  Sum1/1 -> Sum2/1
  FB Gain/1 -> Sum2/2
  FB Gain1/1 -> Product1/2
  Saturation4/1 -> FB Gain1/1
  FmVAS/1 -> FB Gain/1
  OLdxThigh [N]/1 -> Saturation4/1
  Product1/1 -> Sum1/1
  Stimulation Bias/1 -> Sum1/2
  Sum2/1 -> Sum14/1
  Sum14/1 -> StimVAS/1
  Gain2/1 -> Sum14/2
  CLKneeState/1 -> Gain2/1
  OLonCL/1 -> Product1/1

== system nmm2DFullBody/Full Body Control (created using the nmc library)/Subsystem/Parameter variation/Alpha variation/Alpha Variation ==
  alpha : EnablePort  ShowOutputPort=on
  Gain : Gain  Gain=10
  Gain1 : Gain  Gain=0.1
  Ramp : simulink/Sources/Ramp  slope=0.05  start=2  X0=0
  Rounding Function : Rounding  Operator=round
  Saturation : Saturate  UpperLimit=1  LowerLimit=0
  Switch : Switch  Threshold=1
  "alphaOut " : Outport
  wires:
  Switch/1 -> "alphaOut "/1
  Ramp/1 -> Gain/1
  alpha/1 -> Switch/2, Switch/3
  Saturation/1 -> Switch/1
  Gain/1 -> Rounding Function/1
  Rounding Function/1 -> Gain1/1
  Gain1/1 -> Saturation/1

== system nmm2DFullBody/Full Body Control (created using the nmc library)/Subsystem/Parameter variation/Alpha variation/Alpha Variation1 ==
  alpha : EnablePort  ShowOutputPort=on
  Gain : Gain  Gain=10
  Gain1 : Gain  Gain=0.1
  Ramp : simulink/Sources/Ramp  slope=0.05  start=2  X0=0
  Rounding Function : Rounding  Operator=round
  Saturation : Saturate  UpperLimit=1  LowerLimit=0
  Switch : Switch  Threshold=1
  "alphaOut " : Outport
  wires:
  Switch/1 -> "alphaOut "/1
  Ramp/1 -> Gain/1
  alpha/1 -> Switch/2, Switch/3
  Saturation/1 -> Switch/1
  Gain/1 -> Rounding Function/1
  Rounding Function/1 -> Gain1/1
  Gain1/1 -> Saturation/1

== system nmm2DFullBody/Full Body Control (created using the nmc library)/Subsystem/Parameter variation/Alpha variation/Alpha Variation2 ==
  alpha : EnablePort  ShowOutputPort=on
  Gain : Gain  Gain=10
  Gain1 : Gain  Gain=0.1
  Ramp : simulink/Sources/Ramp  slope=0.05  start=2  X0=0
  Rounding Function : Rounding  Operator=round
  Saturation : Saturate  UpperLimit=1  LowerLimit=0
  Switch : Switch  Threshold=1
  "alphaOut " : Outport
  wires:
  Switch/1 -> "alphaOut "/1
  Ramp/1 -> Gain/1
  alpha/1 -> Switch/2, Switch/3
  Saturation/1 -> Switch/1
  Gain/1 -> Rounding Function/1
  Rounding Function/1 -> Gain1/1
  Gain1/1 -> Saturation/1

== system nmm2DFullBody/Full Body Control (created using the nmc library)/Subsystem/Parameter variation/Alpha variation/Alpha Variation3 ==
  alpha : EnablePort  ShowOutputPort=on
  Gain : Gain  Gain=10
  Gain1 : Gain  Gain=0.1
  Ramp : simulink/Sources/Ramp  slope=0.05  start=2  X0=0
  Rounding Function : Rounding  Operator=round
  Saturation : Saturate  UpperLimit=1  LowerLimit=0
  Switch : Switch  Threshold=1
  "alphaOut " : Outport
  wires:
  Switch/1 -> "alphaOut "/1
  Ramp/1 -> Gain/1
  alpha/1 -> Switch/2, Switch/3
  Saturation/1 -> Switch/1
  Gain/1 -> Rounding Function/1
  Rounding Function/1 -> Gain1/1
  Gain1/1 -> Saturation/1

== system nmm2DFullBody/Full Body Control (created using the nmc library)/Subsystem/Parameter variation/Alpha variation/Alpha Variation4 ==
  alpha : EnablePort  ShowOutputPort=on
  Gain : Gain  Gain=10
  Gain1 : Gain  Gain=0.1
  Ramp : simulink/Sources/Ramp  slope=0.05  start=2  X0=0
  Rounding Function : Rounding  Operator=round
  Saturation : Saturate  UpperLimit=1  LowerLimit=0
  Switch : Switch  Threshold=1
  "alphaOut " : Outport
  wires:
  Switch/1 -> "alphaOut "/1
  Ramp/1 -> Gain/1
  alpha/1 -> Switch/2, Switch/3
  Saturation/1 -> Switch/1
  Gain/1 -> Rounding Function/1
  Rounding Function/1 -> Gain1/1
  Gain1/1 -> Saturation/1

== system nmm2DFullBody/Full Body Control (created using the nmc library)/Subsystem/Parameter variation/Alpha variation/Alpha Variation5 ==
  alpha : EnablePort  ShowOutputPort=on
  Gain : Gain  Gain=10
  Gain1 : Gain  Gain=0.1
  Ramp : simulink/Sources/Ramp  slope=0.05  start=2  X0=0
  Rounding Function : Rounding  Operator=round
  Saturation : Saturate  UpperLimit=1  LowerLimit=0
  Switch : Switch  Threshold=1
  "alphaOut " : Outport
  wires:
  Switch/1 -> "alphaOut "/1
  Ramp/1 -> Gain/1
  alpha/1 -> Switch/2, Switch/3
  Saturation/1 -> Switch/1
  Gain/1 -> Rounding Function/1
  Rounding Function/1 -> Gain1/1
  Gain1/1 -> Saturation/1

== system nmm2DFullBody/Full Body Control (created using the nmc library)/Subsystem/Parameter variation/Alpha variation/Alpha Variation6 ==
  alpha : EnablePort  ShowOutputPort=on
  Gain : Gain  Gain=10
  Gain1 : Gain  Gain=0.1
  Ramp : simulink/Sources/Ramp  slope=0.05  start=2  X0=0
  Rounding Function : Rounding  Operator=round
  Saturation : Saturate  UpperLimit=1  LowerLimit=0
  Switch : Switch  Threshold=1
  "alphaOut " : Outport
  wires:
  Switch/1 -> "alphaOut "/1
  Ramp/1 -> Gain/1
  alpha/1 -> Switch/2, Switch/3
  Saturation/1 -> Switch/1
  Gain/1 -> Rounding Function/1
  Rounding Function/1 -> Gain1/1
  Gain1/1 -> Saturation/1

== system nmm2DFullBody/Full Body Control (created using the nmc library)/Subsystem/Parameter variation/Alpha variation/Alpha Variation7 ==
  alpha : EnablePort  ShowOutputPort=on
  Gain : Gain  Gain=10
  Gain1 : Gain  Gain=0.1
  Ramp : simulink/Sources/Ramp  slope=0.05  start=2  X0=0
  Rounding Function : Rounding  Operator=round
  Saturation : Saturate  UpperLimit=1  LowerLimit=0
  Switch : Switch  Threshold=1
  "alphaOut " : Outport
  wires:
  Switch/1 -> "alphaOut "/1
  Ramp/1 -> Gain/1
  alpha/1 -> Switch/2, Switch/3
  Saturation/1 -> Switch/1
  Gain/1 -> Rounding Function/1
  Rounding Function/1 -> Gain1/1
  Gain1/1 -> Saturation/1

== system nmm2DFullBody/Full Body Control (created using the nmc library)/Subsystem/Parameter variation/Alpha variation/Alpha Variation8 ==
  alpha : EnablePort  ShowOutputPort=on
  Gain : Gain  Gain=10
  Gain1 : Gain  Gain=0.1
  Ramp : simulink/Sources/Ramp  slope=0.05  start=2  X0=0
  Rounding Function : Rounding  Operator=round
  Saturation : Saturate  UpperLimit=1  LowerLimit=0
  Switch : Switch  Threshold=1
  "alphaOut " : Outport
  wires:
  Switch/1 -> "alphaOut "/1
  Ramp/1 -> Gain/1
  alpha/1 -> Switch/2, Switch/3
  Saturation/1 -> Switch/1
  Gain/1 -> Rounding Function/1
  Rounding Function/1 -> Gain1/1
  Gain1/1 -> Saturation/1

== system nmm2DFullBody/Full Body Control (created using the nmc library)/Subsystem/Parameter variation/Amplitude Variation/Down ==
  Amp : Inport
  Enable : EnablePort
  Gain : Gain  Gain=10
  Gain1 : Gain  Gain=0.1
  Ramp : simulink/Sources/Ramp  slope=0.04  start=2  X0=0
  Rounding Function : Rounding  Operator=round
  Saturation : Saturate  UpperLimit=1.5  LowerLimit=0
  Subtract : Sum  Inputs=+-
  "AmpDown " : Outport
  wires:
  Saturation/1 -> Subtract/2
  Ramp/1 -> Gain/1
  Amp/1 -> Subtract/1
  Gain/1 -> Rounding Function/1
  Rounding Function/1 -> Gain1/1
  Gain1/1 -> Saturation/1
  Subtract/1 -> "AmpDown "/1

== system nmm2DFullBody/Full Body Control (created using the nmc library)/Subsystem/Parameter variation/Amplitude Variation/Off  ==
  Amp : Inport
  Enable : EnablePort
  "Amp " : Outport
  wires:
  Amp/1 -> "Amp "/1
